simulink model "VPD_lab_4_nonlinear"  (R2022b)
settings: Solver=VariableStepAuto  StartTime=0.0  StopTime=50  RelTol=1e-3
undefined symbols (not defined in the file): B, goal_x, goal_y, J, K1, K2, ke, km, L, r, R, start_x, start_y
settings Model: Creator=Alex  LastModifiedBy=anton
settings SolverCC: ZeroCrossAlgorithm=Adaptive
settings DebuggingCC: MaskedZcDiagnostic=none  IgnoredZcDiagnostic=none

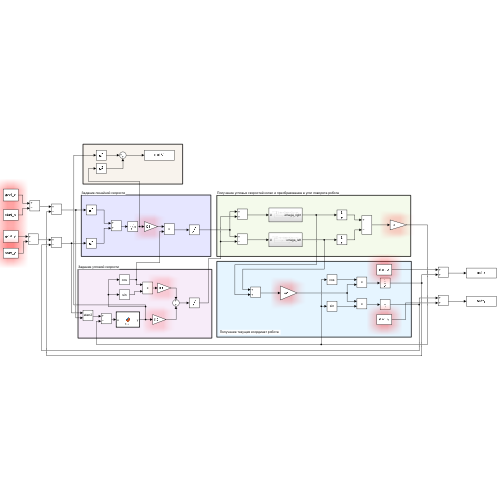
[thumbnail: Simulink's stored preview of the top-level diagram]
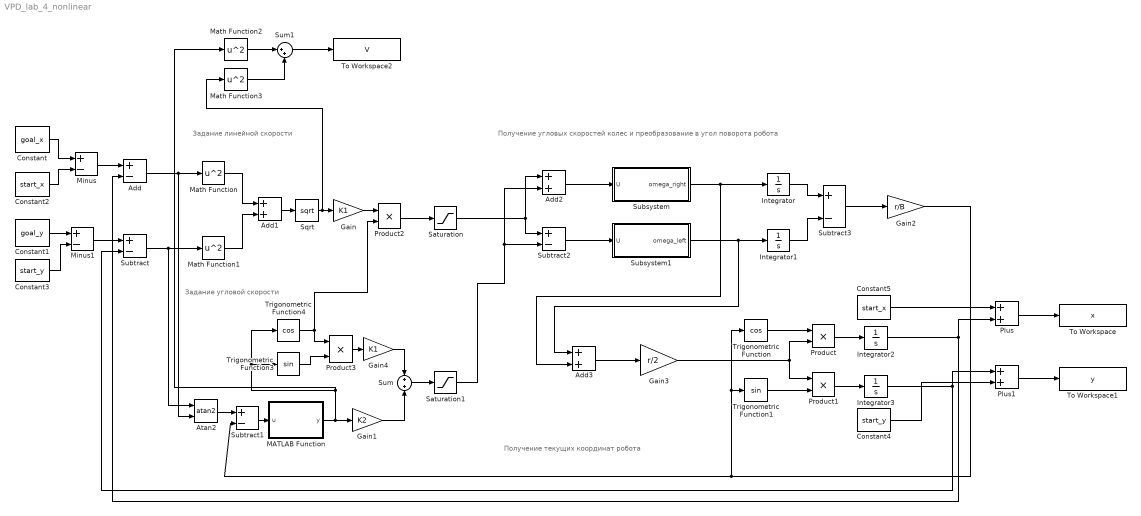
== system VPD_lab_4_nonlinear ==
  note: Получение текущих координат робота
  note: Получение угловых скоростей колес и преобразование в угол поворота робота
  note: Задание угловой скорости
  note: Задание линейной скорости
  Add : Sum  Inputs=+-
  Add1 : Sum
  Add2 : Sum
  Add3 : Sum
  Atan2 : Trigonometry  Operator=atan2
  Constant : Constant  Value=goal_x
  Constant1 : Constant  Value=goal_y
  Constant2 : Constant  Value=start_x
  Constant3 : Constant  Value=start_y
  Constant4 : Constant  Value=start_y
  Constant5 : Constant  Value=start_x
  Gain : Gain  Gain=K1
  Gain1 : Gain  Gain=K2
  Gain2 : Gain  Gain=r/B
  Gain3 : Gain  Gain=r/2
  Gain4 : Gain  Gain=K1
  Integrator{,1..3} (4 alike) : Integrator
  MATLAB Function : MATLAB Function  TreatAsAtomicUnit=on
  Math Function{,1..3} (4 alike) : Math  Operator=square
  Minus : Sum  Inputs=+-
  Minus1 : Sum  Inputs=+-
  Plus : Sum
  Plus1 : Sum
  Product{,1..3} (4 alike) : Product
  Saturation : Saturate  UpperLimit=6.4  LowerLimit=-6.4
  Saturation1 : Saturate  UpperLimit=1.6  LowerLimit=-1.6
  Sqrt : Sqrt
  Subsystem : Subsystem
  Subsystem1 : Subsystem
  Subtract{,1..3} (4 alike) : Sum  Inputs=+-
  Sum : Sum  Inputs=+|+
  Sum1 : Sum  Inputs=|++
  To Workspace : ToWorkspace  VariableName=x  SaveFormat=Timeseries  SampleTime=-1
  To Workspace1 : ToWorkspace  VariableName=y  SaveFormat=Timeseries  SampleTime=-1
  To Workspace2 : ToWorkspace  VariableName=V  SaveFormat=Timeseries  SampleTime=-1
  Trigonometric Function : Trigonometry  Operator=cos
  Trigonometric Function1 : Trigonometry
  Trigonometric Function3 : Trigonometry
  Trigonometric Function4 : Trigonometry  Operator=cos
  wires:
  Subsystem/1(omega_right) -> Integrator/1, Add3/2
  Saturation/1 -> Add2/1, Subtract2/1
  Integrator1/1 -> Subtract3/2
  Subtract2/1 -> Subsystem1/1(U)
  Integrator2/1 -> Add/2, Plus/2
  Gain2/1 -> Subtract1/2, Trigonometric Function1/1, Trigonometric Function/1
  Add1/1 -> Sqrt/1
  Trigonometric Function/1 -> Product/1
  Saturation1/1 -> Subtract2/2, Add2/2
  Add2/1 -> Subsystem/1(U)
  Product1/1 -> Integrator3/1
  Atan2/1 -> Subtract1/1
  Math Function/1 -> Add1/1
  Add3/1 -> Gain3/1
  Integrator3/1 -> Plus1/1, Subtract/2
  Gain3/1 -> Product1/1, Product/2
  Integrator/1 -> Subtract3/1
  Trigonometric Function1/1 -> Product1/2
  Subtract3/1 -> Gain2/1
  Subtract1/1 -> MATLAB Function/1(u)
  MATLAB Function/1(y) -> Trigonometric Function4/1, Trigonometric Function3/1, Math Function2/1, Gain1/1
  Product/1 -> Integrator2/1
  Math Function1/1 -> Add1/2
  Sqrt/1 -> Math Function3/1, Gain/1
  Add/1 -> Atan2/2, Math Function/1
  Subsystem1/1(omega_left) -> Add3/1, Integrator1/1
  Subtract/1 -> Math Function1/1, Atan2/1
  Product2/1 -> Saturation/1
  Gain1/1 -> Sum/2
  Sum/1 -> Saturation1/1
  Trigonometric Function4/1 -> Product3/1, Product2/2
  Trigonometric Function3/1 -> Product3/2
  Product3/1 -> Gain4/1
  Gain4/1 -> Sum/1
  Gain/1 -> Product2/1
  Sum1/1 -> To Workspace2/1
  Math Function2/1 -> Sum1/1
  Math Function3/1 -> Sum1/2
  Constant1/1 -> Minus1/1
  Constant3/1 -> Minus1/2
  Minus1/1 -> Subtract/1
  Constant2/1 -> Minus/2
  Constant/1 -> Minus/1
  Constant5/1 -> Plus/1
  Constant4/1 -> Plus1/2
  Plus1/1 -> To Workspace1/1
  Plus/1 -> To Workspace/1
  Minus/1 -> Add/1

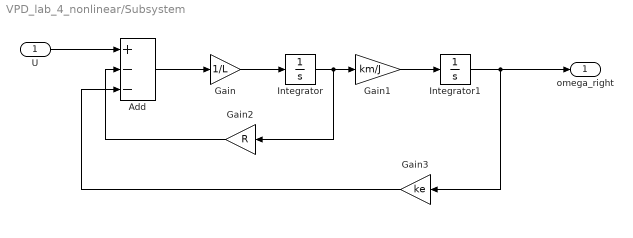
== system VPD_lab_4_nonlinear/Subsystem ==
  U : Inport
  Add : Sum  Inputs=+--
  Gain : Gain  Gain=1/L
  Gain1 : Gain  Gain=km/J
  Gain2 : Gain  Gain=R
  Gain3 : Gain  Gain=ke
  Integrator : Integrator
  Integrator1 : Integrator
  omega_right : Outport
  wires:
  Gain/1 -> Integrator/1
  Integrator1/1 -> Gain3/1, omega_right/1
  Add/1 -> Gain/1
  Gain2/1 -> Add/2
  Integrator/1 -> Gain2/1, Gain1/1
  Gain1/1 -> Integrator1/1
  Gain3/1 -> Add/3
  U/1 -> Add/1

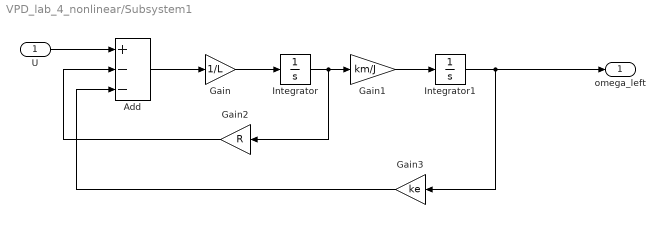
== system VPD_lab_4_nonlinear/Subsystem1 ==
  U : Inport
  Add : Sum  Inputs=+--
  Gain : Gain  Gain=1/L
  Gain1 : Gain  Gain=km/J
  Gain2 : Gain  Gain=R
  Gain3 : Gain  Gain=ke
  Integrator : Integrator
  Integrator1 : Integrator
  omega_left : Outport
  wires:
  U/1 -> Add/1
  Add/1 -> Gain/1
  Gain/1 -> Integrator/1
  Integrator/1 -> Gain2/1, Gain1/1
  Gain2/1 -> Add/2
  Gain1/1 -> Integrator1/1
  Integrator1/1 -> omega_left/1, Gain3/1
  Gain3/1 -> Add/3

== matlab function VPD_lab_4_nonlinear/MATLAB Function ==
  data: u input; y output
function y = fcn(u)
if (u <=-pi)
    y=u+2*pi;
elseif (u>=pi)
    y=u-2*pi;
else
    y=u;
end
